simulink model "sldemo_antiwindupactuator"  (Simulink 7.6)
settings: Solver=ode45  StartTime=0.0  StopTime=200  RelTol=1e-5
libraries: simulink x1
settings Model: Creator=The MathWorks Inc.
settings DebuggingCC: SolverPrmCheckMsg=none

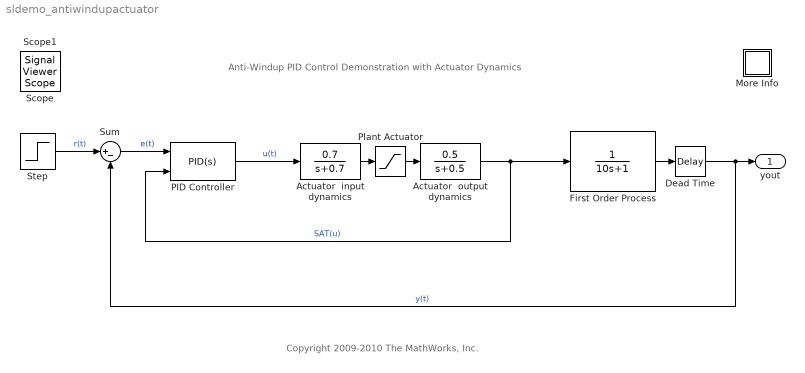
== system sldemo_antiwindupactuator ==
  note: Anti-Windup PID Control Demonstration
      | with Actuator Dynamics
  note: Copyright 2009-2010 The MathWorks, Inc.
  Actuator  input dynamics : TransferFcn  Numerator=[0.7]  Denominator=[1 0.7]
  Actuator  output dynamics : TransferFcn  Numerator=[0.5]  Denominator=[1 0.5]
  Dead Time : TransportDelay  DelayTime=2  BufferSize=2048
  First Order Process : TransferFcn  Numerator=1  Denominator=[10 1]
  More Info : Subsystem
      settings: OpenFcn=showdemo('sldemo_antiwindup')
      mask Display: disp('?')
  PID Controller : simulink/Continuous/PID Controller  DialogController=pidpack.PIDConfig.pidDDGCreate  DialogControllerArgs=DataTag0  SystemSampleTime=-1  Controller=PID  TimeDomain=Continuous-time  SampleTime=1  IntegratorMethod=Forward Euler  FilterMethod=Forward Euler  Form=Parallel  P=1.7018012505578  I=0.208461637073455  D=-1.26102994076046  N=0.178109803713032  InitialConditionSource=internal  InitialConditionForIntegrator=0  InitialConditionForFilter=0  ExternalReset=none  LimitOutput=off  UpperSaturationLimit=10  LowerSaturationLimit=-10  LinearizeAsGain=off  AntiWindupMode=none  Kb=1  TrackingMode=on  Kt=1  PParamMin=[]  PParamMax=[]  IParamMin=[]  IParamMax=[]  DParamMin=[]  DParamMax=[]  NParamMin=[]  NParamMax=[]  KbParamMin=[]  KbParamMax=[]  KtParamMin=[]  KtParamMax=[]  POutMin=[]  POutMax=[]  IOutMin=[]  IOutMax=[]  DOutMin=[]  DOutMax=[]  NOutMin=[]  NOutMax=[]  KbOutMin=[]  KbOutMax=[]  KtOutMin=[]  KtOutMax=[]  IntegratorOutMin=[]  IntegratorOutMax=[]  FilterOutMin=[]  FilterOutMax=[]  SumOutMin=[]  SumOutMax=[]  SumI1OutMin=[]  SumI1OutMax=[]  SumI2OutMin=[]  SumI2OutMax=[]  SumI3OutMin=[]  SumI3OutMax=[]  SumDOutMin=[]  SumDOutMax=[]  SaturationOutMin=[]  SaturationOutMax=[]  IntegratorContinuousStateAttributes=''  IntegratorStateMustResolveToSignalObject=off  IntegratorRTWStateStorageClass=Auto  FilterContinuousStateAttributes=''  FilterStateMustResolveToSignalObject=off  FilterRTWStateStorageClass=Auto
  Plant Actuator : Saturate  UpperLimit=10  LowerLimit=-10
  Step : Step  Time=80  Before=10  After=5  SampleTime=0
  Sum : Sum  Inputs=|+-
  yout : Outport
  Scope : SignalViewerScope  IOType=viewer  LegendLocations="367.3333      228.3333            72            36"  RefreshTime=0.035000
      settings: ShowLegends=on  TimeRange=200  YMin=-2  YMax=12  MaxDataPoints=100000
  Scope1 : SignalViewerScope  IOType=viewer  LegendLocations="345.3333      228.3333            91            36"  RefreshTime=0.035000
      settings: ShowLegends=on  TimeRange=200  YMin=0  YMax=30  MaxDataPoints=100000
  wires:
  Step/1 -> Sum/1  "r(t)"
  Sum/1 -> PID Controller/1  "e(t)"
  Dead Time/1 -> yout/1, Sum/2  "y(t)"
  First Order Process/1 -> Dead Time/1
  Plant Actuator/1 -> Actuator  output dynamics/1
  Actuator  output dynamics/1 -> First Order Process/1, PID Controller/2  "SAT(u)"
  Actuator  input dynamics/1 -> Plant Actuator/1
  PID Controller/1 -> Actuator  input dynamics/1  "u(t)"

== system sldemo_antiwindupactuator/More Info ==
